simulink model "sg_pixel_cnt"  (Simulink 8.2)
settings: Solver=VariableStepDiscrete  StartTime=0.0  StopTime=3*Npxl-1  RelTol=1e-3
values from neighbouring files (symbols this model uses):
  ImgStrmIn = ImgIn'    [tb_pixel_cnt.m]
  ImgX = 640    [tb_pixel_blank_ML_xsvi_inout_only.m]    (also in tb_pixel_cnt.m = SizeI(2))
  ImgY = 480    [tb_pixel_blank_ML_xsvi_inout_only.m]    (also in tb_pixel_cnt.m = SizeI(1))
  Npxl = ImgY * ImgX    (= 307200)    [tb_pixel_blank_ML_xsvi_inout_only.m]    (also in tb_pixel_cnt.m = ImgY * ImgX)
  Radius_ROM = Radius'    [tb_pixel_cnt.m]
libraries: xbsIndex_r4 x17, dspsrcs4 x3
settings Model: Creator=sps  LastModifiedBy=tawassne
settings OptimizationCC: InitFltsAndDblsToZero=on
settings DebuggingCC: SaveWithParameterizedLinksMsg=none  SignalResolutionControl=TryResolveAllWithWarning  SolverPrmCheckMsg=none  MultiTaskDSMMsg=warning  MultiTaskCondExecSysMsg=none
settings RTWCC: IncludeERTFirstTime=on
settings GRTTargetCC: TargetFcnLib=ansi_tfl_tmw.mat

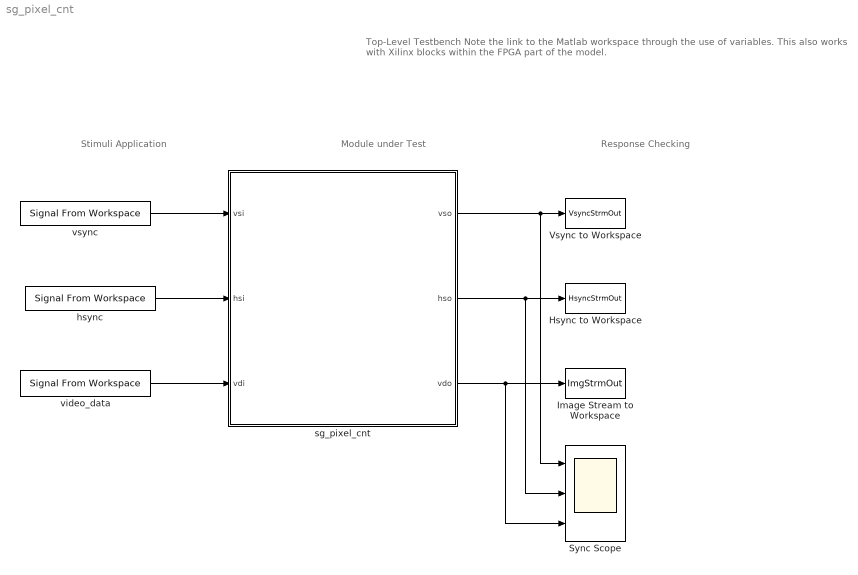
== system sg_pixel_cnt ==
  note: Top-Level Testbench
      | Note the link to the Matlab workspace through the use of variables.
      | This also works with Xilinx blocks within the FPGA part of the model.
  note: Stimuli Application
  note: Response Checking
  note: Module under Test
  Hsync to Workspace : ToWorkspace  VariableName=HsyncStrmOut  SampleTime=-1
      settings: MaxDataPoints=2*Npxl
  Image Stream to Workspace : ToWorkspace  VariableName=ImgStrmOut  SampleTime=-1
      settings: MaxDataPoints=2*Npxl
  Sync Scope : Scope  NumInputPorts=3
      settings: YMin=-5~-5~-5  YMax=5~5~5
  Vsync to Workspace : ToWorkspace  VariableName=VsyncStrmOut  SampleTime=-1
      settings: MaxDataPoints=2*Npxl
  hsync : dspsrcs4/Signal From Workspace  X=[ zeros(1,ImgX-1) 1 ]  Ts=1  nsamps=1  OutputAfterFinalValue=Cyclic repetition  ignoreOrWarnInputAndFrameLengths=off
  sg_pixel_cnt : Subsystem
  video_data : dspsrcs4/Signal From Workspace  X=[ ImgStrmIn(:) ]  Ts=1  nsamps=1  OutputAfterFinalValue=Cyclic repetition  ignoreOrWarnInputAndFrameLengths=off
  vsync : dspsrcs4/Signal From Workspace  X=[ zeros(1,Npxl-1) 1 ]  Ts=1  nsamps=1  OutputAfterFinalValue=Cyclic repetition  ignoreOrWarnInputAndFrameLengths=off
  wires:
  vsync/1 -> sg_pixel_cnt/1(vsi)
  hsync/1 -> sg_pixel_cnt/2(hsi)
  video_data/1 -> sg_pixel_cnt/3(vdi)
  sg_pixel_cnt/1(vso) -> Vsync to Workspace/1, Sync Scope/1
  sg_pixel_cnt/2(hso) -> Hsync to Workspace/1, Sync Scope/2
  sg_pixel_cnt/3(vdo) -> Image Stream to Workspace/1, Sync Scope/3

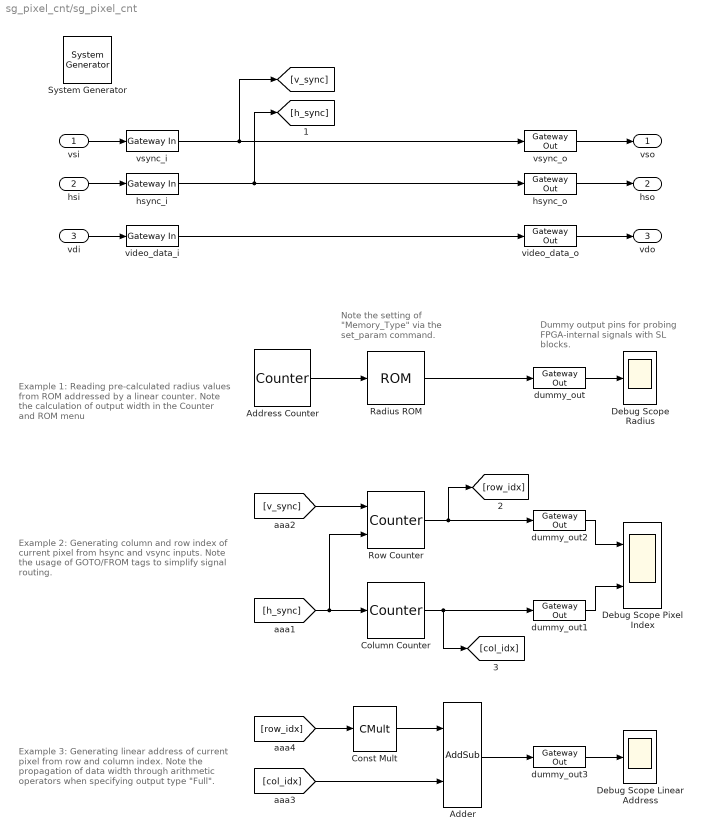
== system sg_pixel_cnt/sg_pixel_cnt ==
  note: Example 1:
      | Reading pre-calculated radius
      | values from ROM addressed by
      | a linear counter.
      | Note the calculation of output width
      | in the Counter and ROM menu
  note: Example 2:
      | Generating column and row index of
      | current pixel from hsync and vsync
      | inputs.
      | Note the usage of GOTO/FROM tags
      | to simplify signal routing.
  note: Example 3:
      | Generating linear address of current
      | pixel from row and column index.
      | Note the propagation of data width
      | through arithmetic operators when
      | specifying output type "Full".
  note: Dummy output pins for
      | probing FPGA-internal
      | signals with SL blocks.
  note: Note the setting of
      | "Memory_Type" via the
      | set_param command.
  vsi : Inport
  hsi : Inport  Port=2
  vdi : Inport  Port=3
  " System Generator" : xbsIndex_r4/ System Generator  Tag=genX  xilinxfamily=spartan6  part=xc6slx150t  speed=-3  package=fgg676  synthesis_tool=XST  clock_wrapper=Clock Enables  directory=./netlist  proj_type=Project Navigator  Synth_file=XST Defaults  Impl_file=ISE Defaults  testbench=off  simulink_period=1  sysclk_period=10  dcm_input_clock_period=10  incr_netlist=off  trim_vbits=Everywhere in SubSystem  dbl_ovrd=According to Block Masks  core_generation=According to Block Masks  run_coregen=off  deprecated_control=off  eval_field=0  block_type=sysgen
      settings: block_version=11.4
  Adder : xbsIndex_r4/AddSub  mode=Addition  use_carryin=off  use_carryout=off  en=off  latency=0  precision=Full  arith_type=Unsigned  n_bits=16  bin_pt=14  quantization=Truncate  overflow=Wrap  dbl_ovrd=off  use_behavioral_HDL=off  hw_selection=Fabric  pipelined=off  block_type=addsub
  Address Counter : xbsIndex_r4/Counter  cnt_type=Count Limited  cnt_to=Npxl-1  operation=Up  start_count=0  cnt_by_val=1  arith_type=Unsigned  n_bits=ceil(log2(Npxl))  bin_pt=0  load_pin=off  rst=off  en=off  explicit_period=on  period=1  dbl_ovrd=off  use_behavioral_HDL=off  implementation=Fabric  block_type=counter
  Column Counter : xbsIndex_r4/Counter  cnt_type=Count Limited  cnt_to=ImgX-1  operation=Up  start_count=0  cnt_by_val=1  arith_type=Unsigned  n_bits=ceil(log2(ImgX))  bin_pt=0  load_pin=off  rst=on  en=off  explicit_period=on  period=1  dbl_ovrd=off  use_behavioral_HDL=off  implementation=Fabric  block_type=counter
  Const Mult : xbsIndex_r4/CMult  const=ImgX  gui_display_data_type=Fixed-point  const_n_bits=ceil(log2(ImgX+1))  const_bin_pt=0  float_type=Single  exp_bits=8  fraction_bits=24  en=off  latency=0  precision=Full  arith_type="Signed  (2's comp)"  n_bits=16  bin_pt=14  quantization=Truncate  overflow=Wrap  dbl_ovrd=off  use_behavioral_HDL=off  mem_type=Distributed RAM  pipeline=off  block_type=cmult
  Debug Scope Linear Address : Scope
      settings: SaveName=ScopeData3
  Debug Scope Pixel Index : Scope  NumInputPorts=2
      settings: YMin=-5~-5  YMax=5~5  SaveName=ScopeData2
  Debug Scope Radius : Scope
  Radius ROM : xbsIndex_r4/ROM  depth=Npxl  initVector=Radius_ROM  distributed_mem=Block RAM  rst=off  init_reg=0  en=off  latency=1  gui_display_data_type=Fixed-point  arith_type=Unsigned  n_bits=ceil(log2(max(max(Radius_ROM)))) + 5  bin_pt=5  preci_type=Single  exp_width=8  frac_width=24  dbl_ovrd=off  optimize=Area  use_rpm=on  block_type=sprom
  Row Counter : xbsIndex_r4/Counter  cnt_type=Count Limited  cnt_to=ImgY-1  operation=Up  start_count=0  cnt_by_val=1  arith_type=Unsigned  n_bits=ceil(log2(ImgY))  bin_pt=0  load_pin=off  rst=on  en=on  explicit_period=on  period=1  dbl_ovrd=off  use_behavioral_HDL=off  implementation=Fabric  block_type=counter
  dummy_out{,1..3} (4 alike) : xbsIndex_r4/Gateway Out  hdl_port=off  timing_constraint=None  locs_specified=off  LOCs={}  block_type=gatewayout
      settings: infoedit="Gateway out block.  Converts Xilinx fixed point or floating-point type inputs into ouputs of type Simulink integer, double, or fixed point.<br><br>Hardware notes:  In hardware these blocks become top level output ports or are discarded, depending on how they are configured."  xl_area=[0, 0, 0, 0, 0, 0, 0]  block_version=VER_STRING_GOES_HERE
  hsync_i : xbsIndex_r4/Gateway In  gui_display_data_type=Fixed-point  arith_type=Boolean  n_bits=1  bin_pt=0  preci_type=Single  exp_width=8  frac_width=24  quantization="Round  (unbiased: +/- Inf)"  overflow=Saturate  period=1  dbl_ovrd=off  timing_constraint=None  locs_specified=off  LOCs={}  hdl_port=on  block_type=gatewayin
      settings: infoedit="Gateway in block.  Converts inputs of type Simulink integer, double and fixed point to  Xilinx fixed point type.<br><br>Hardware notes:  In hardware these blocks become top level input ports."  xl_area=[0, 0, 0, 0, 0, 0, 0]  block_version=VER_STRING_GOES_HERE
  hsync_o : xbsIndex_r4/Gateway Out  hdl_port=on  timing_constraint=None  locs_specified=off  LOCs={}  block_type=gatewayout
      settings: infoedit="Gateway out block.  Converts Xilinx fixed point inputs into ouputs of type Simulink integer, double, or fixed point.<P><P>Hardware notes:  In hardware these blocks become top level output ports or are discarded, depending on how they are configured."  xl_area=[0, 0, 0, 0, 0, 0, 0]  block_version=VER_STRING_GOES_HERE
  video_data_i : xbsIndex_r4/Gateway In  gui_display_data_type=Fixed-point  arith_type=Unsigned  n_bits=8  bin_pt=0  preci_type=Single  exp_width=8  frac_width=24  quantization="Round  (unbiased: +/- Inf)"  overflow=Saturate  period=1  dbl_ovrd=off  timing_constraint=None  locs_specified=off  LOCs={}  hdl_port=on  block_type=gatewayin
      settings: infoedit="Gateway in block.  Converts inputs of type Simulink integer, double and fixed point to  Xilinx fixed point type.<br><br>Hardware notes:  In hardware these blocks become top level input ports."  xl_area=[0, 0, 0, 0, 0, 0, 0]  block_version=VER_STRING_GOES_HERE
  video_data_o : xbsIndex_r4/Gateway Out  hdl_port=on  timing_constraint=None  locs_specified=off  LOCs={}  block_type=gatewayout
      settings: infoedit="Gateway out block.  Converts Xilinx fixed point or floating-point type inputs into ouputs of type Simulink integer, double, or fixed point.<br><br>Hardware notes:  In hardware these blocks become top level output ports or are discarded, depending on how they are configured."  xl_area=[0, 0, 0, 0, 0, 0, 0]  block_version=VER_STRING_GOES_HERE
  vsync_i : xbsIndex_r4/Gateway In  gui_display_data_type=Fixed-point  arith_type=Boolean  n_bits=1  bin_pt=0  preci_type=Single  exp_width=8  frac_width=24  quantization="Round  (unbiased: +/- Inf)"  overflow=Saturate  period=1  dbl_ovrd=off  timing_constraint=None  locs_specified=off  LOCs={}  hdl_port=on  block_type=gatewayin
      settings: infoedit="Gateway in block.  Converts inputs of type Simulink integer, double and fixed point to  Xilinx fixed point type.<br><br>Hardware notes:  In hardware these blocks become top level input ports."  xl_area=[0, 0, 0, 0, 0, 0, 0]  block_version=VER_STRING_GOES_HERE
  vsync_o : xbsIndex_r4/Gateway Out  hdl_port=on  timing_constraint=None  locs_specified=off  LOCs={}  block_type=gatewayout
      settings: infoedit="Gateway out block.  Converts Xilinx fixed point inputs into ouputs of type Simulink integer, double, or fixed point.<P><P>Hardware notes:  In hardware these blocks become top level output ports or are discarded, depending on how they are configured."  xl_area=[0, 0, 0, 0, 0, 0, 0]  block_version=VER_STRING_GOES_HERE
  vso : Outport
  hso : Outport  Port=2
  vdo : Outport  Port=3
  wires:
  vdi/1 -> video_data_i/1
  video_data_o/1 -> vdo/1
  vsi/1 -> vsync_i/1
  hsi/1 -> hsync_i/1
  vsync_o/1 -> vso/1
  hsync_o/1 -> hso/1
  video_data_i/1 -> video_data_o/1
  vsync_i/1 -> vsync_o/1, [v_sync]
  hsync_i/1 -> hsync_o/1, [h_sync]
  Address Counter/1 -> Radius ROM/1
  Radius ROM/1 -> dummy_out/1
  dummy_out/1 -> Debug Scope Radius/1
  [h_sync] -> Column Counter/1, Row Counter/2
  Column Counter/1 -> dummy_out1/1, [col_idx]
  Row Counter/1 -> dummy_out2/1, [row_idx]
  [v_sync] -> Row Counter/1
  dummy_out2/1 -> Debug Scope Pixel Index/1
  dummy_out1/1 -> Debug Scope Pixel Index/2
  [row_idx] -> Const Mult/1
  Const Mult/1 -> Adder/1
  [col_idx] -> Adder/2
  Adder/1 -> dummy_out3/1
  dummy_out3/1 -> Debug Scope Linear Address/1
